simulink model "spm1"  (Simulink 3.00)
settings: Solver=ode45  SolverMode=SingleTasking  StartTime=0.0  StopTime=999999  MaxStep=10  RelTol=1e-3  AbsTol=1e-6
settings Model: SaveTime=off  SaveOutput=off

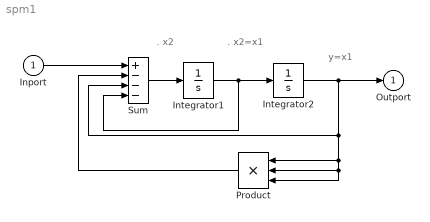
== system spm1 ==
  note: .
      | x2
  note: y=x1
  note: .
      | x2=x1
  Inport : Inport  Port=1  PortWidth=-1  SampleTime=-1  DataType=auto
      settings: SignalType=auto
  Integrator1 : Integrator  ExternalReset=none  InitialConditionSource=internal  InitialCondition=0  LimitOutput=off  UpperSaturationLimit=inf  LowerSaturationLimit=-inf  ShowSaturationPort=off  ShowStatePort=off  AbsoluteTolerance=auto
  Integrator2 : Integrator  ExternalReset=none  InitialConditionSource=internal  InitialCondition=0  LimitOutput=off  UpperSaturationLimit=inf  LowerSaturationLimit=-inf  ShowSaturationPort=off  ShowStatePort=off  AbsoluteTolerance=auto
  Product : Product  Orientation=left  Inputs=3  SaturateOnIntegerOverflow=on
  Sum : Sum  Inputs=+---  SaturateOnIntegerOverflow=on
  Outport : Outport  Port=1
  wires:
  Sum/1 -> Integrator1/1
  Product/1 -> Sum/2
  Integrator1/1 -> Sum/4, Integrator2/1
  Integrator2/1 -> Product/1, Product/2, Product/3, Sum/3, Outport/1
  Inport/1 -> Sum/1
